simulink model "schema_filtre_IIR"  (R2017b)
settings: Solver=VariableStepAuto  StartTime=0.0  StopTime=10.0  RelTol=1e-3
values from neighbouring files (symbols this model uses):
  a1 = 2*cos(teta)    [generation_signal.m]
  a2 = -1    [generation_signal.m]
undefined symbols (not defined in the file or in its folder): a0, b0, b1, b2
settings Model: Creator=laure  LastModifiedBy=laure

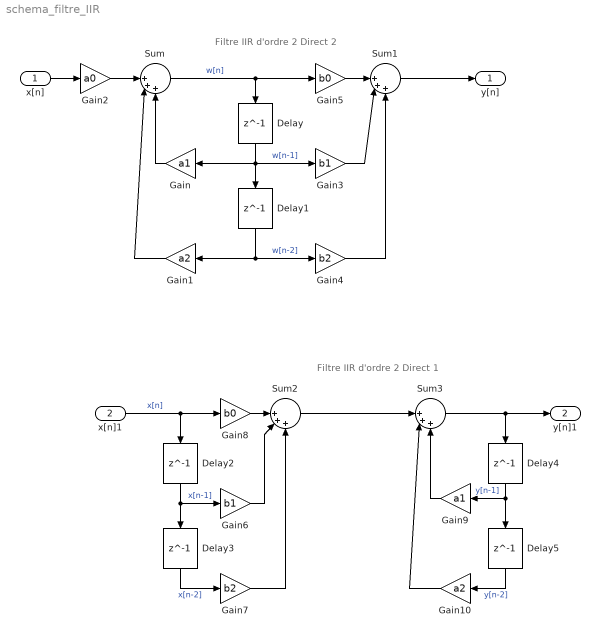
== system schema_filtre_IIR ==
  note: Filtre IIR d'ordre 2
      | Direct 2
  note: Filtre IIR d'ordre 2
      | Direct 1
  x[n] : Inport
  x[n]1 : Inport  Port=2
  Delay{,1..5} (6 alike) : Delay  DelayLength=1  InitialCondition=0
  Gain : Gain  Gain=a1
  Gain1 : Gain  Gain=a2
  Gain10 : Gain  Gain=a2
  Gain2 : Gain  Gain=a0
  Gain3 : Gain  Gain=b1
  Gain4 : Gain  Gain=b2
  Gain5 : Gain  Gain=b0
  Gain6 : Gain  Gain=b1
  Gain7 : Gain  Gain=b2
  Gain8 : Gain  Gain=b0
  Gain9 : Gain  Gain=a1
  Sum{,1..3} (4 alike) : Sum  Inputs=||+++
  y[n] : Outport
  y[n]1 : Outport  Port=2
  wires:
  Delay/1 -> Gain/1, Gain3/1, Delay1/1  "w[n-1]"
  x[n]/1 -> Gain2/1
  Gain2/1 -> Sum/1
  Delay1/1 -> Gain4/1, Gain1/1  "w[n-2]"
  Gain/1 -> Sum/3
  Gain1/1 -> Sum/2
  Sum/1 -> Gain5/1, Delay/1  "w[n]"
  Gain5/1 -> Sum1/1
  Gain3/1 -> Sum1/2
  Gain4/1 -> Sum1/3
  Sum1/1 -> y[n]/1
  Sum3/1 -> Delay4/1, y[n]1/1
  x[n]1/1 -> Delay2/1, Gain8/1  "x[n]"
  Gain8/1 -> Sum2/1
  Delay3/1 -> Gain7/1  "x[n-2]"
  Delay2/1 -> Gain6/1, Delay3/1  "x[n-1]"
  Gain6/1 -> Sum2/2
  Gain7/1 -> Sum2/3
  Delay4/1 -> Gain9/1, Delay5/1  "y[n-1]"
  Delay5/1 -> Gain10/1  "y[n-2]"
  Sum2/1 -> Sum3/1
  Gain9/1 -> Sum3/3
  Gain10/1 -> Sum3/2
